simulink model "DCOM6"  (Simulink 7.8)
settings: Solver=ode45  StartTime=0.0  StopTime=10.0  RelTol=1e-3
settings Model: Creator=DJSCE.Student  LastModifiedBy=DJSCE.Student

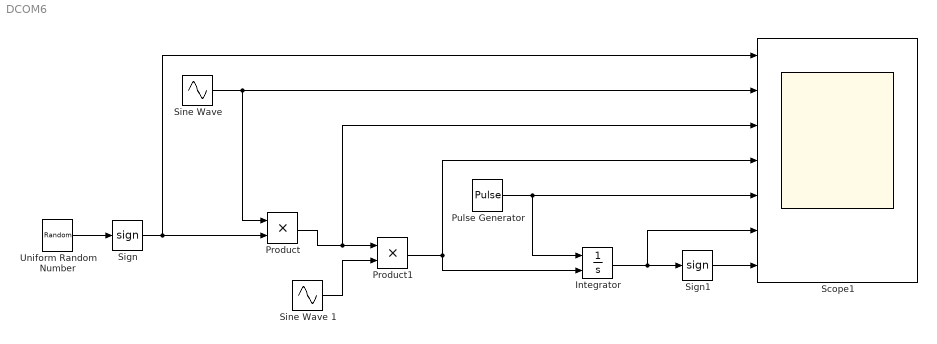
== system DCOM6 ==
  Integrator : Integrator  ExternalReset=rising
  Product : Product  RndMeth=Zero
  Product1 : Product  RndMeth=Zero
  Pulse Generator : DiscretePulseGenerator  PulseType=Time based  Period=1  PulseWidth=5
  Scope1 : Scope  NumInputPorts=7
      settings: TimeRange=11  YMin=-2~-5~-5~-5~-2~-2~-2  YMax=2~5~5~5~2~2~2
  Sign : Signum
  Sign1 : Signum
  Sine Wave : Sin  Frequency=2*pi  SampleTime=0.001
  Sine Wave 1 : Sin  Frequency=2*pi  SampleTime=0.001
  Uniform Random Number : UniformRandomNumber  SampleTime=1
  wires:
  Uniform Random Number/1 -> Sign/1
  Sine Wave 1/1 -> Product1/2
  Product/1 -> Product1/1, Scope1/3
  Integrator/1 -> Sign1/1, Scope1/6
  Sign1/1 -> Scope1/7
  Product1/1 -> Integrator/2, Scope1/4
  Pulse Generator/1 -> Integrator/1, Scope1/5
  Sign/1 -> Product/2, Scope1/1
  Sine Wave/1 -> Scope1/2, Product/1
